simulink model "d2cTest"  (Simulink 7.9)
settings: Solver=ode45  StartTime=0.0  StopTime=100  RelTol=1e-3
settings Model: Creator=MAR  LastModifiedBy=MAR

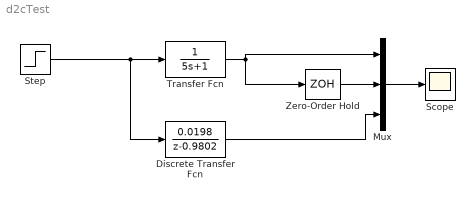
== system d2cTest ==
  Discrete Transfer Fcn : DiscreteTransferFcn  Numerator=[0.0198]  Denominator=[1 -0.9802]  SampleTime=0.1
  Mux : Mux  Inputs=3
  Scope : Scope
  Step : Step  SampleTime=0
  Transfer Fcn : TransferFcn  Denominator=[5 1]
  Zero-Order Hold : ZeroOrderHold  SampleTime=0.1
  wires:
  Transfer Fcn/1 -> Zero-Order Hold/1, Mux/1
  Step/1 -> Transfer Fcn/1, Discrete Transfer Fcn/1
  Mux/1 -> Scope/1
  Zero-Order Hold/1 -> Mux/2
  Discrete Transfer Fcn/1 -> Mux/3
